simulink model "rst_simulink"  (R2022b)
settings: Solver=VariableStepAuto  StartTime=0.0  StopTime=10.0  RelTol=1e-3
values from neighbouring files (symbols this model uses):
  q0 = [0;0;q_thumb;q_index;q_mid;q_ring;q_little]    [create_Hand_Model_wt_Muscles.m]    (also in create_MSK_Mojtaba.m = zeros(Mojtaba_hand.nj,1))
libraries: robotmaniplib x3
settings Model: Creator=ge26jow  LastModifiedBy=ge26jow

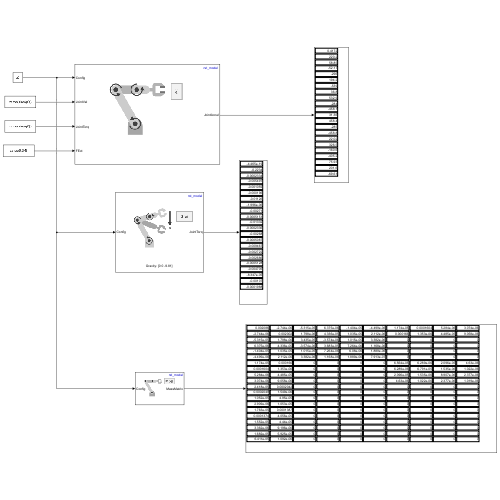
[thumbnail: Simulink's stored preview of the top-level diagram]
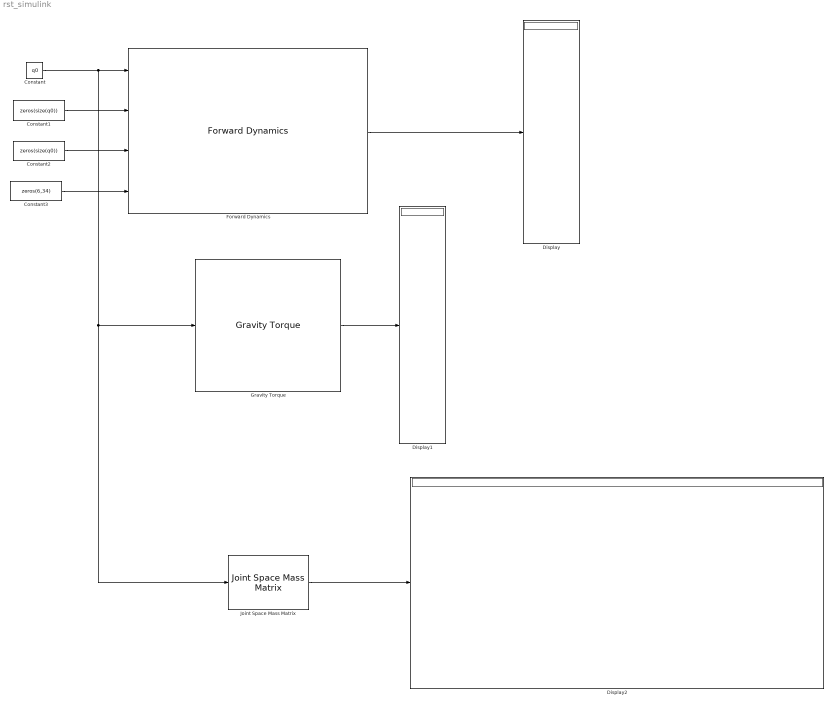
== system rst_simulink ==
  Constant : Constant  Value=q0
  Constant1 : Constant  Value=zeros(size(q0))
  Constant2 : Constant  Value=zeros(size(q0))
  Constant3 : Constant  Value=zeros(6,34)
  Display : Display
  Display1 : Display
  Display2 : Display
  Forward Dynamics : robotmaniplib/Forward Dynamics  RigidBodyTree=rst_model  SimulateUsing=Interpreted execution
  Gravity Torque : robotmaniplib/Gravity Torque  RigidBodyTree=rst_model  SimulateUsing=Interpreted execution
  Joint Space Mass Matrix : robotmaniplib/Joint Space Mass Matrix  RigidBodyTree=rst_model  SimulateUsing=Interpreted execution
  wires:
  Constant/1 -> Joint Space Mass Matrix/1, Gravity Torque/1, Forward Dynamics/1
  Constant1/1 -> Forward Dynamics/2
  Constant2/1 -> Forward Dynamics/3
  Constant3/1 -> Forward Dynamics/4
  Forward Dynamics/1 -> Display/1
  Gravity Torque/1 -> Display1/1
  Joint Space Mass Matrix/1 -> Display2/1
